simulink model "SDT_Roboticarm_UR5_motion_comparison"  (R2020b)
settings: Solver=VariableStepAuto  StartTime=0.0  StopTime=10.0  RelTol=1e-3
undefined symbols (not defined in the file or in its folder): chaser, InvDyn, ureal, uss
libraries: SDTlibV1 x12, RCTblocks x9
settings Model: Creator=T.FORMOSA  LastModifiedBy=ricardorodrigues
settings DebuggingCC: AlgebraicLoopMsg=none  ArithmeticOperatorsInVariantConditions=warning
settings SFSimCC: CustomCodeUndefinedFunction=UseInterfaceOnly

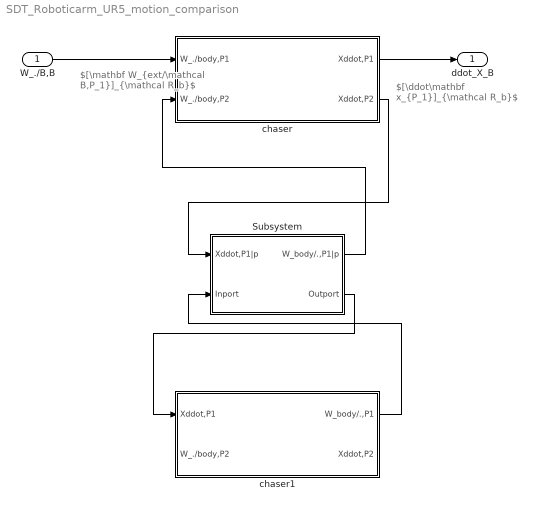
== system SDT_Roboticarm_UR5_motion_comparison ==
  note: $[\mathbf W_{ext/\mathcal B,P_1}]_{\mathcal R_b}$
  note: $[\ddot\mathbf x_{P_1}]_{\mathcal R_b}$
  W_./B,B : Inport
  Subsystem : Subsystem
  chaser : Subsystem  mask(Multi-port rigid body (6nx6n)){m=chaser.rigidhub.wetmass, Ig=chaser.rigidhub.inertias, OG=[0;0;0], n=2, numinv=none, OP1=[0;0;0], OP2=[0;0;chaser.rigidhub.height/2], OP3=[ureal('P3_y',1,'percent',10);0;0], OP4=[0;0;0], OP5=[0;0;0]}
      mask prompts: m "Mass (Kg)"; Ig "Inertia (at G, Kg m^2)"; OG "OG (3x1 vector, m)"; n "Number of ports"; numinv "Port to be inverted"; OP1 "OP1 (3x1 vector, m)"; OP2 "OP2 (3x1 vector, m)"; OP3 "OP3 (3x1 vector, m)"; OP4 "OP4 (3x1 vector, m)"; OP5 "OP5 (3x1 vector,m)"
      mask help:
      | 6nx6n inverse dynamic model between:
      |    *  wrenches applied to this body at the given n points,
      |    * acceleration twiists at he n given points.
      |
      | The 6x6 channel asociated to a single given point can be inverted
      mask init:
      | MultiPortRigidBody
      mask Help: web('Docmultiportrigidbody.html')
      mask TypeOptions n: 1 | 2 | 3 | 4 | 5
      mask TypeOptions numinv: none | 1 | 2 | 3 | 4 | 5
      mask DialogControl Control1 Prompt: Inverse Dynamic model of a rigid body at n given points (ports):
      mask DialogControl Control2 Prompt: 6nx6n transfer between wrenches applied at the n points and accelaretion twists at these points
      mask DialogControl Control3 Prompt: 0: the reference point
      mask DialogControl Control4 Prompt: G: the center of mass
      mask DialogControl Control5 Prompt: Pi (i=1:n): the n given connection points (n<6).
      mask DialogControl Control6 Prompt: All parameters are expressed in the body frame.
      mask DialogControl Control7 Prompt: Each parameter can be an uncertain parameter declared with "ureal"
      mask DialogControl Control8 Prompt: The 6x6 channel associated to one port can be inverted: then the input of this channel is the acceleration twist imposed at this point and the output is the wrench applied by this body.
      mask DialogControl ParameterGroupVar Prompt: Main parameters
      mask DialogControl port1 Prompt: Port #1
      mask DialogControl port2 Prompt: #2
      mask DialogControl port3 Prompt: #3
      mask DialogControl port4 Prompt: #4
      mask DialogControl port5 Prompt: #5
      mask Display:
      | disp('Multi-port\n rigid body\n (6nx6n)')
      | if n==1,
      |     if numinv-1==1,
      |         port_label('input', 1,'Xddot,P')
      |         port_label('output',1,'W_body/.,P')
      |     else
      |         port_label('input', 1,'W_./body,P')
      |         port_label('output',1,'Xddot,P')
      |     end
      | else
      |     for ii=1:n
      |         if numinv==ii+1,
      |             port_label('output',ii,['W_body/.,P',num2str(ii)])
      |             port_label('input', ii,['Xddot,P',num2str(ii)])
      |         else
      |             port_label('input', ii,['W_./body,P',num2str(ii)])
      |             port_label('output',ii,['Xddot,P',num2str(ii)])
      |         end
      |     end
      | end
  chaser1 : Subsystem  mask(Multi-port rigid body (6nx6n)){m=chaser.rigidhub.wetmass, Ig=chaser.rigidhub.inertias, OG=[0;0;0], n=2, numinv=1, OP1=[0;0;0], OP2=[0;0;chaser.rigidhub.height/2], OP3=[ureal('P3_y',1,'percent',10);0;0], OP4=[0;0;0], OP5=[0;0;0]}
      mask prompts: m "Mass (Kg)"; Ig "Inertia (at G, Kg m^2)"; OG "OG (3x1 vector, m)"; n "Number of ports"; numinv "Port to be inverted"; OP1 "OP1 (3x1 vector, m)"; OP2 "OP2 (3x1 vector, m)"; OP3 "OP3 (3x1 vector, m)"; OP4 "OP4 (3x1 vector, m)"; OP5 "OP5 (3x1 vector,m)"
      mask help:
      | 6nx6n inverse dynamic model between:
      |    *  wrenches applied to this body at the given n points,
      |    * acceleration twiists at he n given points.
      |
      | The 6x6 channel asociated to a single given point can be inverted
      mask init:
      | MultiPortRigidBody
      mask Help: web('Docmultiportrigidbody.html')
      mask TypeOptions n: 1 | 2 | 3 | 4 | 5
      mask TypeOptions numinv: none | 1 | 2 | 3 | 4 | 5
      mask DialogControl Control1 Prompt: Inverse Dynamic model of a rigid body at n given points (ports):
      mask DialogControl Control2 Prompt: 6nx6n transfer between wrenches applied at the n points and accelaretion twists at these points
      mask DialogControl Control3 Prompt: 0: the reference point
      mask DialogControl Control4 Prompt: G: the center of mass
      mask DialogControl Control5 Prompt: Pi (i=1:n): the n given connection points (n<6).
      mask DialogControl Control6 Prompt: All parameters are expressed in the body frame.
      mask DialogControl Control7 Prompt: Each parameter can be an uncertain parameter declared with "ureal"
      mask DialogControl Control8 Prompt: The 6x6 channel associated to one port can be inverted: then the input of this channel is the acceleration twist imposed at this point and the output is the wrench applied by this body.
      mask DialogControl ParameterGroupVar Prompt: Main parameters
      mask DialogControl port1 Prompt: Port #1
      mask DialogControl port2 Prompt: #2
      mask DialogControl port3 Prompt: #3
      mask DialogControl port4 Prompt: #4
      mask DialogControl port5 Prompt: #5
      mask Display:
      | disp('Multi-port\n rigid body\n (6nx6n)')
      | if n==1,
      |     if numinv-1==1,
      |         port_label('input', 1,'Xddot,P')
      |         port_label('output',1,'W_body/.,P')
      |     else
      |         port_label('input', 1,'W_./body,P')
      |         port_label('output',1,'Xddot,P')
      |     end
      | else
      |     for ii=1:n
      |         if numinv==ii+1,
      |             port_label('output',ii,['W_body/.,P',num2str(ii)])
      |             port_label('input', ii,['Xddot,P',num2str(ii)])
      |         else
      |             port_label('input', ii,['W_./body,P',num2str(ii)])
      |             port_label('output',ii,['Xddot,P',num2str(ii)])
      |         end
      |     end
      | end
  ddot_X_B : Outport  VectorParamsAs1DForOutWhenUnconnected=off
  wires:
  W_./B,B/1 -> chaser/1(W_./body,P1)
  chaser/1(Xddot,P1) -> ddot_X_B/1
  chaser/2(Xddot,P2) -> Subsystem/1(Xddot,P1|p)
  Subsystem/1(W_body/.,P1|p) -> chaser/2(W_./body,P2)
  Subsystem/2(Outport) -> chaser1/1(Xddot,P1)
  chaser1/1(W_body/.,P1) -> Subsystem/2(Inport)

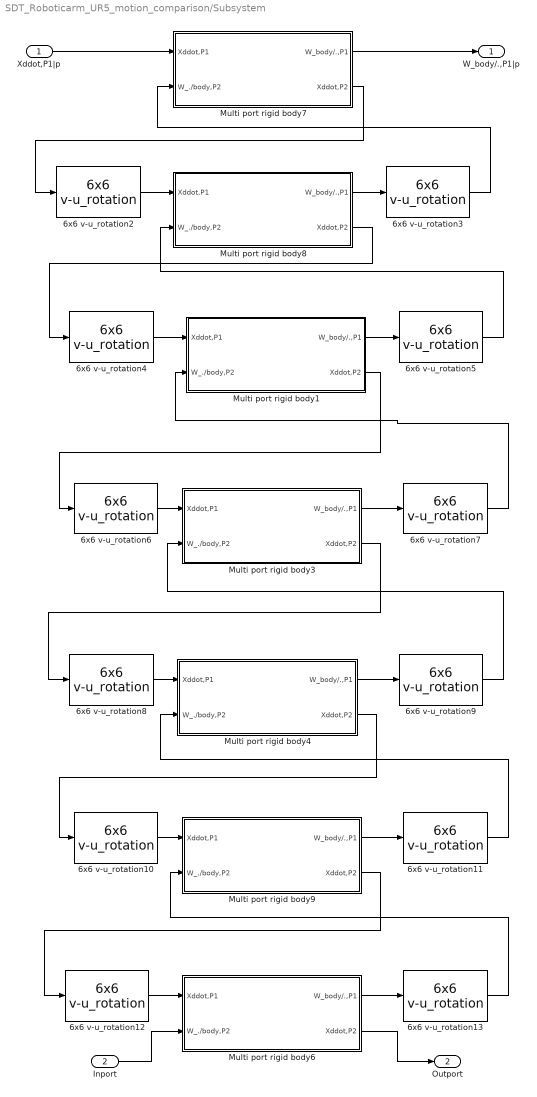
== system SDT_Roboticarm_UR5_motion_comparison/Subsystem ==
  Xddot,P1|p : Inport
  Inport : Inport  Port=2
  6x6 v-u_rotation10 : SDTlibV1/3//6 dof DCM/6x6 v-u_rotation  ra=[0;0;-1]  theta=chaser.robotic_arm_servicing.init_angles(5)  transp=on
  6x6 v-u_rotation11 : SDTlibV1/3//6 dof DCM/6x6 v-u_rotation  ra=[0;0;-1]  theta=chaser.robotic_arm_servicing.init_angles(5)  transp=off
  6x6 v-u_rotation12 : SDTlibV1/3//6 dof DCM/6x6 v-u_rotation  ra=[0;1;0]  theta=chaser.robotic_arm_servicing.init_angles(6)  transp=on
  6x6 v-u_rotation13 : SDTlibV1/3//6 dof DCM/6x6 v-u_rotation  ra=[0;1;0]  theta=chaser.robotic_arm_servicing.init_angles(6)  transp=off
  6x6 v-u_rotation2 : SDTlibV1/3//6 dof DCM/6x6 v-u_rotation  ra=[0;0;1]  theta=chaser.robotic_arm_servicing.init_angles(1)  transp=on
  6x6 v-u_rotation3 : SDTlibV1/3//6 dof DCM/6x6 v-u_rotation  ra=[0;0;1]  theta=chaser.robotic_arm_servicing.init_angles(1)  transp=off
  6x6 v-u_rotation4 : SDTlibV1/3//6 dof DCM/6x6 v-u_rotation  ra=[0;1;0]  theta=chaser.robotic_arm_servicing.init_angles(2)  transp=on
  6x6 v-u_rotation5 : SDTlibV1/3//6 dof DCM/6x6 v-u_rotation  ra=[0;1;0]  theta=chaser.robotic_arm_servicing.init_angles(2)  transp=off
  6x6 v-u_rotation6 : SDTlibV1/3//6 dof DCM/6x6 v-u_rotation  ra=[0;1;0]  theta=chaser.robotic_arm_servicing.init_angles(3)  transp=on
  6x6 v-u_rotation7 : SDTlibV1/3//6 dof DCM/6x6 v-u_rotation  ra=[0;1;0]  theta=chaser.robotic_arm_servicing.init_angles(3)  transp=off
  6x6 v-u_rotation8 : SDTlibV1/3//6 dof DCM/6x6 v-u_rotation  ra=[0;1;0]  theta=chaser.robotic_arm_servicing.init_angles(4)  transp=on
  6x6 v-u_rotation9 : SDTlibV1/3//6 dof DCM/6x6 v-u_rotation  ra=[0;1;0]  theta=chaser.robotic_arm_servicing.init_angles(4)  transp=off
  Multi port rigid body1 : Subsystem  mask(Multi-port rigid body (6nx6n)){m=8.393000000000001, Ig=[0.0151074 0 0;0 0.22689067591 0;0 0 0.22689067591], OG=[0.28;0;0], n=2, numinv=1, OP1=[0;0;0], OP2=[0.425; -0.1197; 0], OP3=[0;0;0], OP4=[0;0;0], OP5=[0;0;0]}
      mask prompts: m "Mass (Kg)"; Ig "Inertia (at G, Kg m^2)"; OG "OG (3x1 vector, m)"; n "Number of ports"; numinv "Port to be inverted"; OP1 "OP1 (3x1 vector, m)"; OP2 "OP2 (3x1 vector, m)"; OP3 "OP3 (3x1 vector, m)"; OP4 "OP4 (3x1 vector, m)"; OP5 "OP5 (3x1 vector,m)"
      mask help:
      | 6nx6n dynamic model of a rigid body at n given points (ports) between wrenches applied at the n points (input) and acceleration twists at these points (output).
      |
      | 0: the reference point
      | G: the center of mass
      | Pi (i=1:n): the n given connection points (n<6).
      |
      | All parameters are expressed in the body frame.
      | Each parameter can be an uncertain parameter declared with "ureal"
      |
      | The 6x6 channel associated to one port can be inverted: then the input of this channel is the acceleration twist imposed at this point and the output is the wrench applied by this body.
      mask init:
      | MultiPortRigidBody
      mask Help: web('Docmultiportrigidbody.html')
      mask TypeOptions n: 1 | 2 | 3 | 4 | 5
      mask TypeOptions numinv: none | 1 | 2 | 3 | 4 | 5
      mask DialogControl ParameterGroupVar Prompt: Main parameters
      mask DialogControl port1 Prompt: Port #1
      mask DialogControl port2 Prompt: #2
      mask DialogControl port3 Prompt: #3
      mask DialogControl port4 Prompt: #4
      mask DialogControl port5 Prompt: #5
      mask Display:
      | disp('Multi-port\n rigid body\n (6nx6n)')
      | if n==1,
      |     if numinv-1==1,
      |         port_label('input', 1,'Xddot,P')
      |         port_label('output',1,'W_body/.,P')
      |     else
      |         port_label('input', 1,'W_./body,P')
      |         port_label('output',1,'Xddot,P')
      |     end
      | else
      |     for ii=1:n
      |         if numinv==ii+1,
      |             port_label('output',ii,['W_body/.,P',num2str(ii)])
      |             port_label('input', ii,['Xddot,P',num2str(ii)])
      |         else
      |             port_label('input', ii,['W_./body,P',num2str(ii)])
      |             port_label('output',ii,['Xddot,P',num2str(ii)])
      |         end
      |     end
      | end
  Multi port rigid body3 : Subsystem  mask(Multi-port rigid body (6nx6n)){m=2.275, Ig=[0.004095 0 0;0 0.049443313556 0;0 0 0.049443313556], OG=[0.25;0;0], n=2, numinv=1, OP1=[0;0;0], OP2=[0.39225; 0; 0], OP3=[0;0;0], OP4=[0;0;0], OP5=[0;0;0]}
      mask prompts: m "Mass (Kg)"; Ig "Inertia (at G, Kg m^2)"; OG "OG (3x1 vector, m)"; n "Number of ports"; numinv "Port to be inverted"; OP1 "OP1 (3x1 vector, m)"; OP2 "OP2 (3x1 vector, m)"; OP3 "OP3 (3x1 vector, m)"; OP4 "OP4 (3x1 vector, m)"; OP5 "OP5 (3x1 vector,m)"
      mask help:
      | 6nx6n dynamic model of a rigid body at n given points (ports) between wrenches applied at the n points (input) and acceleration twists at these points (output).
      |
      | 0: the reference point
      | G: the center of mass
      | Pi (i=1:n): the n given connection points (n<6).
      |
      | All parameters are expressed in the body frame.
      | Each parameter can be an uncertain parameter declared with "ureal"
      |
      | The 6x6 channel associated to one port can be inverted: then the input of this channel is the acceleration twist imposed at this point and the output is the wrench applied by this body.
      mask init:
      | MultiPortRigidBody
      mask Help: web('Docmultiportrigidbody.html')
      mask TypeOptions n: 1 | 2 | 3 | 4 | 5
      mask TypeOptions numinv: none | 1 | 2 | 3 | 4 | 5
      mask DialogControl ParameterGroupVar Prompt: Main parameters
      mask DialogControl port1 Prompt: Port #1
      mask DialogControl port2 Prompt: #2
      mask DialogControl port3 Prompt: #3
      mask DialogControl port4 Prompt: #4
      mask DialogControl port5 Prompt: #5
      mask Display:
      | disp('Multi-port\n rigid body\n (6nx6n)')
      | if n==1,
      |     if numinv-1==1,
      |         port_label('input', 1,'Xddot,P')
      |         port_label('output',1,'W_body/.,P')
      |     else
      |         port_label('input', 1,'W_./body,P')
      |         port_label('output',1,'Xddot,P')
      |     end
      | else
      |     for ii=1:n
      |         if numinv==ii+1,
      |             port_label('output',ii,['W_body/.,P',num2str(ii)])
      |             port_label('input', ii,['Xddot,P',num2str(ii)])
      |         else
      |             port_label('input', ii,['W_./body,P',num2str(ii)])
      |             port_label('output',ii,['Xddot,P',num2str(ii)])
      |         end
      |     end
      | end
  Multi port rigid body4 : Subsystem  mask(Multi-port rigid body (6nx6n)){m=1.219, Ig=[0.111172755531 0 0;0 0.111172755531 0;0 0 0.21942], OG=[0;0;0], n=2, numinv=1, OP1=[0;0;0], OP2=[0; 0.093; 0], OP3=[0;0;0], OP4=[0;0;0], OP5=[0;0;0]}
      mask prompts: m "Mass (Kg)"; Ig "Inertia (at G, Kg m^2)"; OG "OG (3x1 vector, m)"; n "Number of ports"; numinv "Port to be inverted"; OP1 "OP1 (3x1 vector, m)"; OP2 "OP2 (3x1 vector, m)"; OP3 "OP3 (3x1 vector, m)"; OP4 "OP4 (3x1 vector, m)"; OP5 "OP5 (3x1 vector,m)"
      mask help:
      | 6nx6n dynamic model of a rigid body at n given points (ports) between wrenches applied at the n points (input) and acceleration twists at these points (output).
      |
      | 0: the reference point
      | G: the center of mass
      | Pi (i=1:n): the n given connection points (n<6).
      |
      | All parameters are expressed in the body frame.
      | Each parameter can be an uncertain parameter declared with "ureal"
      |
      | The 6x6 channel associated to one port can be inverted: then the input of this channel is the acceleration twist imposed at this point and the output is the wrench applied by this body.
      mask init:
      | MultiPortRigidBody
      mask Help: web('Docmultiportrigidbody.html')
      mask TypeOptions n: 1 | 2 | 3 | 4 | 5
      mask TypeOptions numinv: none | 1 | 2 | 3 | 4 | 5
      mask DialogControl ParameterGroupVar Prompt: Main parameters
      mask DialogControl port1 Prompt: Port #1
      mask DialogControl port2 Prompt: #2
      mask DialogControl port3 Prompt: #3
      mask DialogControl port4 Prompt: #4
      mask DialogControl port5 Prompt: #5
      mask Display:
      | disp('Multi-port\n rigid body\n (6nx6n)')
      | if n==1,
      |     if numinv-1==1,
      |         port_label('input', 1,'Xddot,P')
      |         port_label('output',1,'W_body/.,P')
      |     else
      |         port_label('input', 1,'W_./body,P')
      |         port_label('output',1,'Xddot,P')
      |     end
      | else
      |     for ii=1:n
      |         if numinv==ii+1,
      |             port_label('output',ii,['W_body/.,P',num2str(ii)])
      |             port_label('input', ii,['Xddot,P',num2str(ii)])
      |         else
      |             port_label('input', ii,['W_./body,P',num2str(ii)])
      |             port_label('output',ii,['Xddot,P',num2str(ii)])
      |         end
      |     end
      | end
  Multi port rigid body6 : Subsystem  mask(Multi-port rigid body (6nx6n)){m=0.1879, Ig=[0.0171364731454 0 0;0 0.0171364731454 0;0 0 0.033822], OG=[0;0;0], n=2, numinv=1, OP1=[0;0;0], OP2=[0; 0.0823; 0], OP3=[0;0;0], OP4=[0;0;0], OP5=[0;0;0]}
      mask prompts: m "Mass (Kg)"; Ig "Inertia (at G, Kg m^2)"; OG "OG (3x1 vector, m)"; n "Number of ports"; numinv "Port to be inverted"; OP1 "OP1 (3x1 vector, m)"; OP2 "OP2 (3x1 vector, m)"; OP3 "OP3 (3x1 vector, m)"; OP4 "OP4 (3x1 vector, m)"; OP5 "OP5 (3x1 vector,m)"
      mask help:
      | 6nx6n dynamic model of a rigid body at n given points (ports) between wrenches applied at the n points (input) and acceleration twists at these points (output).
      |
      | 0: the reference point
      | G: the center of mass
      | Pi (i=1:n): the n given connection points (n<6).
      |
      | All parameters are expressed in the body frame.
      | Each parameter can be an uncertain parameter declared with "ureal"
      |
      | The 6x6 channel associated to one port can be inverted: then the input of this channel is the acceleration twist imposed at this point and the output is the wrench applied by this body.
      mask init:
      | MultiPortRigidBody
      mask Help: web('Docmultiportrigidbody.html')
      mask TypeOptions n: 1 | 2 | 3 | 4 | 5
      mask TypeOptions numinv: none | 1 | 2 | 3 | 4 | 5
      mask DialogControl ParameterGroupVar Prompt: Main parameters
      mask DialogControl port1 Prompt: Port #1
      mask DialogControl port2 Prompt: #2
      mask DialogControl port3 Prompt: #3
      mask DialogControl port4 Prompt: #4
      mask DialogControl port5 Prompt: #5
      mask Display:
      | disp('Multi-port\n rigid body\n (6nx6n)')
      | if n==1,
      |     if numinv-1==1,
      |         port_label('input', 1,'Xddot,P')
      |         port_label('output',1,'W_body/.,P')
      |     else
      |         port_label('input', 1,'W_./body,P')
      |         port_label('output',1,'Xddot,P')
      |     end
      | else
      |     for ii=1:n
      |         if numinv==ii+1,
      |             port_label('output',ii,['W_body/.,P',num2str(ii)])
      |             port_label('input', ii,['Xddot,P',num2str(ii)])
      |         else
      |             port_label('input', ii,['W_./body,P',num2str(ii)])
      |             port_label('output',ii,['Xddot,P',num2str(ii)])
      |         end
      |     end
      | end
  Multi port rigid body7 : Subsystem  mask(Multi-port rigid body (6nx6n)){m=4, Ig=[0.00443333156 0 0; 0 0.00443333156 0; 0 0 0.0072], OG=[0;0;0], n=2, numinv=1, OP1=[0;0;0], OP2=[0;0;0.089159], OP3=[0;0;0], OP4=[0;0;0], OP5=[0;0;0]}
      mask prompts: m "Mass (Kg)"; Ig "Inertia (at G, Kg m^2)"; OG "OG (3x1 vector, m)"; n "Number of ports"; numinv "Port to be inverted"; OP1 "OP1 (3x1 vector, m)"; OP2 "OP2 (3x1 vector, m)"; OP3 "OP3 (3x1 vector, m)"; OP4 "OP4 (3x1 vector, m)"; OP5 "OP5 (3x1 vector,m)"
      mask help:
      | 6nx6n dynamic model of a rigid body at n given points (ports) between wrenches applied at the n points (input) and acceleration twists at these points (output).
      |
      | 0: the reference point
      | G: the center of mass
      | Pi (i=1:n): the n given connection points (n<6).
      |
      | All parameters are expressed in the body frame.
      | Each parameter can be an uncertain parameter declared with "ureal"
      |
      | The 6x6 channel associated to one port can be inverted: then the input of this channel is the acceleration twist imposed at this point and the output is the wrench applied by this body.
      mask init:
      | MultiPortRigidBody
      mask Help: web('Docmultiportrigidbody.html')
      mask TypeOptions n: 1 | 2 | 3 | 4 | 5
      mask TypeOptions numinv: none | 1 | 2 | 3 | 4 | 5
      mask DialogControl ParameterGroupVar Prompt: Main parameters
      mask DialogControl port1 Prompt: Port #1
      mask DialogControl port2 Prompt: #2
      mask DialogControl port3 Prompt: #3
      mask DialogControl port4 Prompt: #4
      mask DialogControl port5 Prompt: #5
      mask Display:
      | disp('Multi-port\n rigid body\n (6nx6n)')
      | if n==1,
      |     if numinv-1==1,
      |         port_label('input', 1,'Xddot,P')
      |         port_label('output',1,'W_body/.,P')
      |     else
      |         port_label('input', 1,'W_./body,P')
      |         port_label('output',1,'Xddot,P')
      |     end
      | else
      |     for ii=1:n
      |         if numinv==ii+1,
      |             port_label('output',ii,['W_body/.,P',num2str(ii)])
      |             port_label('input', ii,['Xddot,P',num2str(ii)])
      |         else
      |             port_label('input', ii,['W_./body,P',num2str(ii)])
      |             port_label('output',ii,['Xddot,P',num2str(ii)])
      |         end
      |     end
      | end
  Multi port rigid body8 : Subsystem  mask(Multi-port rigid body (6nx6n)){m=3.7, Ig=[0.010267495893 0 0; 0 0.010267495893 0; 0 0 0.00666], OG=[0;0;0], n=2, numinv=1, OP1=[0;0;0], OP2=[0;0.13585;0], OP3=[0;0;0], OP4=[0;0;0], OP5=[0;0;0]}
      mask prompts: m "Mass (Kg)"; Ig "Inertia (at G, Kg m^2)"; OG "OG (3x1 vector, m)"; n "Number of ports"; numinv "Port to be inverted"; OP1 "OP1 (3x1 vector, m)"; OP2 "OP2 (3x1 vector, m)"; OP3 "OP3 (3x1 vector, m)"; OP4 "OP4 (3x1 vector, m)"; OP5 "OP5 (3x1 vector,m)"
      mask help:
      | 6nx6n dynamic model of a rigid body at n given points (ports) between wrenches applied at the n points (input) and acceleration twists at these points (output).
      |
      | 0: the reference point
      | G: the center of mass
      | Pi (i=1:n): the n given connection points (n<6).
      |
      | All parameters are expressed in the body frame.
      | Each parameter can be an uncertain parameter declared with "ureal"
      |
      | The 6x6 channel associated to one port can be inverted: then the input of this channel is the acceleration twist imposed at this point and the output is the wrench applied by this body.
      mask init:
      | MultiPortRigidBody
      mask Help: web('Docmultiportrigidbody.html')
      mask TypeOptions n: 1 | 2 | 3 | 4 | 5
      mask TypeOptions numinv: none | 1 | 2 | 3 | 4 | 5
      mask DialogControl ParameterGroupVar Prompt: Main parameters
      mask DialogControl port1 Prompt: Port #1
      mask DialogControl port2 Prompt: #2
      mask DialogControl port3 Prompt: #3
      mask DialogControl port4 Prompt: #4
      mask DialogControl port5 Prompt: #5
      mask Display:
      | disp('Multi-port\n rigid body\n (6nx6n)')
      | if n==1,
      |     if numinv-1==1,
      |         port_label('input', 1,'Xddot,P')
      |         port_label('output',1,'W_body/.,P')
      |     else
      |         port_label('input', 1,'W_./body,P')
      |         port_label('output',1,'Xddot,P')
      |     end
      | else
      |     for ii=1:n
      |         if numinv==ii+1,
      |             port_label('output',ii,['W_body/.,P',num2str(ii)])
      |             port_label('input', ii,['Xddot,P',num2str(ii)])
      |         else
      |             port_label('input', ii,['W_./body,P',num2str(ii)])
      |             port_label('output',ii,['Xddot,P',num2str(ii)])
      |         end
      |     end
      | end
  Multi port rigid body9 : Subsystem  mask(Multi-port rigid body (6nx6n)){m=1.219, Ig=[0.111172755531 0 0;0 0.111172755531 0;0 0 0.21942], OG=[0;0;0], n=2, numinv=1, OP1=[0;0;0], OP2=[0; 0; -0.09465], OP3=[0;0;0], OP4=[0;0;0], OP5=[0;0;0]}
      mask prompts: m "Mass (Kg)"; Ig "Inertia (at G, Kg m^2)"; OG "OG (3x1 vector, m)"; n "Number of ports"; numinv "Port to be inverted"; OP1 "OP1 (3x1 vector, m)"; OP2 "OP2 (3x1 vector, m)"; OP3 "OP3 (3x1 vector, m)"; OP4 "OP4 (3x1 vector, m)"; OP5 "OP5 (3x1 vector,m)"
      mask help:
      | 6nx6n dynamic model of a rigid body at n given points (ports) between wrenches applied at the n points (input) and acceleration twists at these points (output).
      |
      | 0: the reference point
      | G: the center of mass
      | Pi (i=1:n): the n given connection points (n<6).
      |
      | All parameters are expressed in the body frame.
      | Each parameter can be an uncertain parameter declared with "ureal"
      |
      | The 6x6 channel associated to one port can be inverted: then the input of this channel is the acceleration twist imposed at this point and the output is the wrench applied by this body.
      mask init:
      | MultiPortRigidBody
      mask Help: web('Docmultiportrigidbody.html')
      mask TypeOptions n: 1 | 2 | 3 | 4 | 5
      mask TypeOptions numinv: none | 1 | 2 | 3 | 4 | 5
      mask DialogControl ParameterGroupVar Prompt: Main parameters
      mask DialogControl port1 Prompt: Port #1
      mask DialogControl port2 Prompt: #2
      mask DialogControl port3 Prompt: #3
      mask DialogControl port4 Prompt: #4
      mask DialogControl port5 Prompt: #5
      mask Display:
      | disp('Multi-port\n rigid body\n (6nx6n)')
      | if n==1,
      |     if numinv-1==1,
      |         port_label('input', 1,'Xddot,P')
      |         port_label('output',1,'W_body/.,P')
      |     else
      |         port_label('input', 1,'W_./body,P')
      |         port_label('output',1,'Xddot,P')
      |     end
      | else
      |     for ii=1:n
      |         if numinv==ii+1,
      |             port_label('output',ii,['W_body/.,P',num2str(ii)])
      |             port_label('input', ii,['Xddot,P',num2str(ii)])
      |         else
      |             port_label('input', ii,['W_./body,P',num2str(ii)])
      |             port_label('output',ii,['Xddot,P',num2str(ii)])
      |         end
      |     end
      | end
  W_body/.,P1|p : Outport
  Outport : Outport  Port=2
  wires:
  6x6 v-u_rotation9/1 -> Multi port rigid body3/2(W_./body,P2)
  Multi port rigid body7/1(W_body/.,P1) -> W_body/.,P1|p/1
  Multi port rigid body6/1(W_body/.,P1) -> 6x6 v-u_rotation13/1
  Multi port rigid body8/2(Xddot,P2) -> 6x6 v-u_rotation4/1
  Multi port rigid body1/2(Xddot,P2) -> 6x6 v-u_rotation6/1
  Multi port rigid body4/1(W_body/.,P1) -> 6x6 v-u_rotation9/1
  Multi port rigid body3/1(W_body/.,P1) -> 6x6 v-u_rotation7/1
  Multi port rigid body8/1(W_body/.,P1) -> 6x6 v-u_rotation3/1
  6x6 v-u_rotation13/1 -> Multi port rigid body9/2(W_./body,P2)
  6x6 v-u_rotation4/1 -> Multi port rigid body1/1(Xddot,P1)
  6x6 v-u_rotation3/1 -> Multi port rigid body7/2(W_./body,P2)
  6x6 v-u_rotation5/1 -> Multi port rigid body8/2(W_./body,P2)
  6x6 v-u_rotation8/1 -> Multi port rigid body4/1(Xddot,P1)
  6x6 v-u_rotation6/1 -> Multi port rigid body3/1(Xddot,P1)
  Xddot,P1|p/1 -> Multi port rigid body7/1(Xddot,P1)
  Multi port rigid body9/1(W_body/.,P1) -> 6x6 v-u_rotation11/1
  6x6 v-u_rotation12/1 -> Multi port rigid body6/1(Xddot,P1)
  Multi port rigid body7/2(Xddot,P2) -> 6x6 v-u_rotation2/1
  Multi port rigid body3/2(Xddot,P2) -> 6x6 v-u_rotation8/1
  6x6 v-u_rotation10/1 -> Multi port rigid body9/1(Xddot,P1)
  6x6 v-u_rotation7/1 -> Multi port rigid body1/2(W_./body,P2)
  6x6 v-u_rotation11/1 -> Multi port rigid body4/2(W_./body,P2)
  6x6 v-u_rotation2/1 -> Multi port rigid body8/1(Xddot,P1)
  Multi port rigid body9/2(Xddot,P2) -> 6x6 v-u_rotation12/1
  Multi port rigid body4/2(Xddot,P2) -> 6x6 v-u_rotation10/1
  Multi port rigid body1/1(W_body/.,P1) -> 6x6 v-u_rotation5/1
  Multi port rigid body6/2(Xddot,P2) -> Outport/1
  Inport/1 -> Multi port rigid body6/2(W_./body,P2)

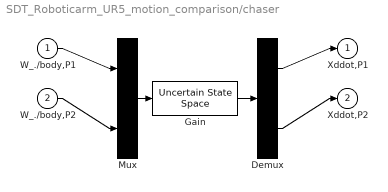
== system SDT_Roboticarm_UR5_motion_comparison/chaser ==
  W_./body,P1 : Inport  PortDimensions=6
  W_./body,P2 : Inport  Port=2  PortDimensions=6
  Demux : Demux  Outputs=[6 6]
      settings: DisplayOption=none
  Gain : RCTblocks/Uncertain State Space  Tag=USS  USystem=uss(InvDyn)  UValue=[]  X0=[]  uX0=[]
      settings: SourceProductBaseCode=RC
  Mux : Mux  Inputs=[6 6]
  Xddot,P1 : Outport  VectorParamsAs1DForOutWhenUnconnected=off
  Xddot,P2 : Outport  Port=2  VectorParamsAs1DForOutWhenUnconnected=off
  wires:
  Mux/1 -> Gain/1
  Gain/1 -> Demux/1
  W_./body,P1/1 -> Mux/1
  Demux/1 -> Xddot,P1/1
  W_./body,P2/1 -> Mux/2
  Demux/2 -> Xddot,P2/1

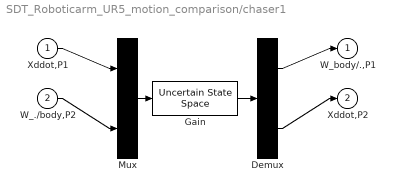
== system SDT_Roboticarm_UR5_motion_comparison/chaser1 ==
  Xddot,P1 : Inport  PortDimensions=6
  W_./body,P2 : Inport  Port=2  PortDimensions=6
  Demux : Demux  Outputs=[6 6]
      settings: DisplayOption=none
  Gain : RCTblocks/Uncertain State Space  Tag=USS  USystem=uss(InvDyn)  UValue=[]  X0=[]  uX0=[]
      settings: SourceProductBaseCode=RC
  Mux : Mux  Inputs=[6 6]
  W_body/.,P1 : Outport  VectorParamsAs1DForOutWhenUnconnected=off
  Xddot,P2 : Outport  Port=2  VectorParamsAs1DForOutWhenUnconnected=off
  wires:
  Mux/1 -> Gain/1
  Gain/1 -> Demux/1
  Xddot,P1/1 -> Mux/1
  Demux/1 -> W_body/.,P1/1
  W_./body,P2/1 -> Mux/2
  Demux/2 -> Xddot,P2/1

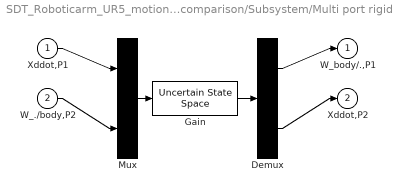
== system SDT_Roboticarm_UR5_motion_comparison/Subsystem/Multi port rigid body1 ==
  Xddot,P1 : Inport  PortDimensions=6
  W_./body,P2 : Inport  Port=2  PortDimensions=6
  Demux : Demux  Outputs=[6 6]
  Gain : RCTblocks/Uncertain State Space  Tag=USS  USystem=uss(InvDyn)  UValue=[]  X0=[]  uX0=[]
      settings: SourceProductBaseCode=RC
  Mux : Mux  Inputs=[6 6]
  W_body/.,P1 : Outport
  Xddot,P2 : Outport  Port=2
  wires:
  Mux/1 -> Gain/1
  Gain/1 -> Demux/1
  Xddot,P1/1 -> Mux/1
  Demux/1 -> W_body/.,P1/1
  W_./body,P2/1 -> Mux/2
  Demux/2 -> Xddot,P2/1

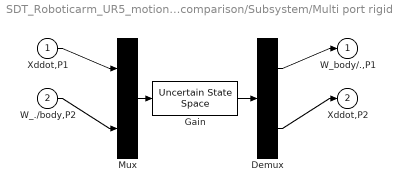
== system SDT_Roboticarm_UR5_motion_comparison/Subsystem/Multi port rigid body3 ==
  Xddot,P1 : Inport  PortDimensions=6
  W_./body,P2 : Inport  Port=2  PortDimensions=6
  Demux : Demux  Outputs=[6 6]
  Gain : RCTblocks/Uncertain State Space  Tag=USS  USystem=uss(InvDyn)  UValue=[]  X0=[]  uX0=[]
      settings: SourceProductBaseCode=RC
  Mux : Mux  Inputs=[6 6]
  W_body/.,P1 : Outport
  Xddot,P2 : Outport  Port=2
  wires:
  Mux/1 -> Gain/1
  Gain/1 -> Demux/1
  Xddot,P1/1 -> Mux/1
  Demux/1 -> W_body/.,P1/1
  W_./body,P2/1 -> Mux/2
  Demux/2 -> Xddot,P2/1

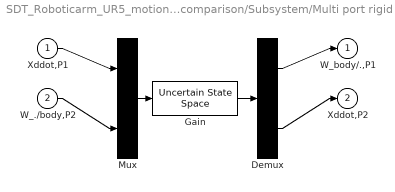
== system SDT_Roboticarm_UR5_motion_comparison/Subsystem/Multi port rigid body4 ==
  Xddot,P1 : Inport  PortDimensions=6
  W_./body,P2 : Inport  Port=2  PortDimensions=6
  Demux : Demux  Outputs=[6 6]
  Gain : RCTblocks/Uncertain State Space  Tag=USS  USystem=uss(InvDyn)  UValue=[]  X0=[]  uX0=[]
      settings: SourceProductBaseCode=RC
  Mux : Mux  Inputs=[6 6]
  W_body/.,P1 : Outport
  Xddot,P2 : Outport  Port=2
  wires:
  Mux/1 -> Gain/1
  Gain/1 -> Demux/1
  Xddot,P1/1 -> Mux/1
  Demux/1 -> W_body/.,P1/1
  W_./body,P2/1 -> Mux/2
  Demux/2 -> Xddot,P2/1

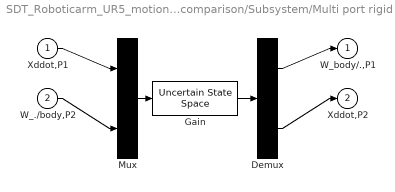
== system SDT_Roboticarm_UR5_motion_comparison/Subsystem/Multi port rigid body6 ==
  Xddot,P1 : Inport  PortDimensions=6
  W_./body,P2 : Inport  Port=2  PortDimensions=6
  Demux : Demux  Outputs=[6 6]
  Gain : RCTblocks/Uncertain State Space  Tag=USS  USystem=uss(InvDyn)  UValue=[]  X0=[]  uX0=[]
      settings: SourceProductBaseCode=RC
  Mux : Mux  Inputs=[6 6]
  W_body/.,P1 : Outport
  Xddot,P2 : Outport  Port=2
  wires:
  Mux/1 -> Gain/1
  Gain/1 -> Demux/1
  Xddot,P1/1 -> Mux/1
  Demux/1 -> W_body/.,P1/1
  W_./body,P2/1 -> Mux/2
  Demux/2 -> Xddot,P2/1

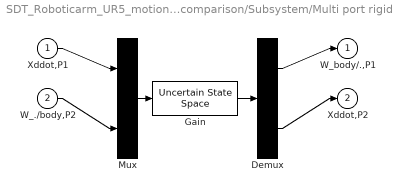
== system SDT_Roboticarm_UR5_motion_comparison/Subsystem/Multi port rigid body7 ==
  Xddot,P1 : Inport  PortDimensions=6
  W_./body,P2 : Inport  Port=2  PortDimensions=6
  Demux : Demux  Outputs=[6 6]
  Gain : RCTblocks/Uncertain State Space  Tag=USS  USystem=uss(InvDyn)  UValue=[]  X0=[]  uX0=[]
      settings: SourceProductBaseCode=RC
  Mux : Mux  Inputs=[6 6]
  W_body/.,P1 : Outport
  Xddot,P2 : Outport  Port=2
  wires:
  Mux/1 -> Gain/1
  Gain/1 -> Demux/1
  Xddot,P1/1 -> Mux/1
  Demux/1 -> W_body/.,P1/1
  W_./body,P2/1 -> Mux/2
  Demux/2 -> Xddot,P2/1

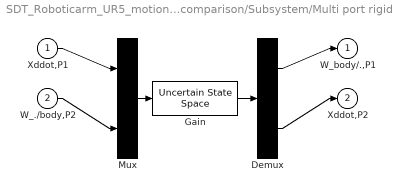
== system SDT_Roboticarm_UR5_motion_comparison/Subsystem/Multi port rigid body8 ==
  Xddot,P1 : Inport  PortDimensions=6
  W_./body,P2 : Inport  Port=2  PortDimensions=6
  Demux : Demux  Outputs=[6 6]
  Gain : RCTblocks/Uncertain State Space  Tag=USS  USystem=uss(InvDyn)  UValue=[]  X0=[]  uX0=[]
      settings: SourceProductBaseCode=RC
  Mux : Mux  Inputs=[6 6]
  W_body/.,P1 : Outport
  Xddot,P2 : Outport  Port=2
  wires:
  Mux/1 -> Gain/1
  Gain/1 -> Demux/1
  Xddot,P1/1 -> Mux/1
  Demux/1 -> W_body/.,P1/1
  W_./body,P2/1 -> Mux/2
  Demux/2 -> Xddot,P2/1

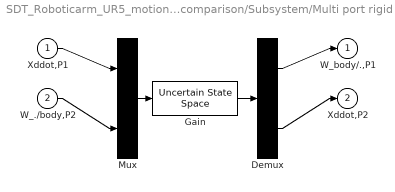
== system SDT_Roboticarm_UR5_motion_comparison/Subsystem/Multi port rigid body9 ==
  Xddot,P1 : Inport  PortDimensions=6
  W_./body,P2 : Inport  Port=2  PortDimensions=6
  Demux : Demux  Outputs=[6 6]
  Gain : RCTblocks/Uncertain State Space  Tag=USS  USystem=uss(InvDyn)  UValue=[]  X0=[]  uX0=[]
      settings: SourceProductBaseCode=RC
  Mux : Mux  Inputs=[6 6]
  W_body/.,P1 : Outport
  Xddot,P2 : Outport  Port=2
  wires:
  Mux/1 -> Gain/1
  Gain/1 -> Demux/1
  Xddot,P1/1 -> Mux/1
  Demux/1 -> W_body/.,P1/1
  W_./body,P2/1 -> Mux/2
  Demux/2 -> Xddot,P2/1
